simulink model "fdm"  (R2023b)
settings: Solver=VariableStepDiscrete  StartTime=0.0  StopTime=0.02  RelTol=1e-3
libraries: commanapbnd3 x3
settings Model: Creator=RomaW11  LastModifiedBy=RomaW11
settings SolverCC: AlgebraicLoopSolver=TrustRegion
settings DataIOCC: LimitDataPoints=on  SaveOutput=off  SaveTime=off
settings OptimizationCC: BooleanDataType=off  DefaultParameterBehavior=Inlined  LocalBlockOutputs=off  LifeSpan=inf
settings DebuggingCC: AlgebraicLoopMsg=error  SingleTaskRateTransMsg=error  UnconnectedInputMsg=warning  UnconnectedOutputMsg=warning  UnconnectedLineMsg=warning  AllowSymbolicDim=off  SFUnexpectedBacktrackingDiag=warning  SFNoUnconditionalDefaultTransitionDiag=warning  SFExecutionAtInitializationDiag=none  ArithmeticOperatorsInVariantConditions=warning
settings ModelReferenceCC: EnableRefExpFcnMdlSchedulingChecks=on
settings SFSimCC: SimUseLocalCustomCode=off  CustomCodeUndefinedFunction=UseInterfaceOnly
settings RTWCC: RTWUseLocalCustomCode=off
settings CodeAppCC: StateflowObjectComments=on
settings GRTTargetCC: TargetLangStandard=C89/C90 (ANSI)
settings ConfigComp: CovMetricSettings=dw  CovSaveCumulativeToWorkspaceVar=on  CovSaveSingleToWorkspaceVar=on  CovExternalEMLEnable=off  CovSFcnEnable=off

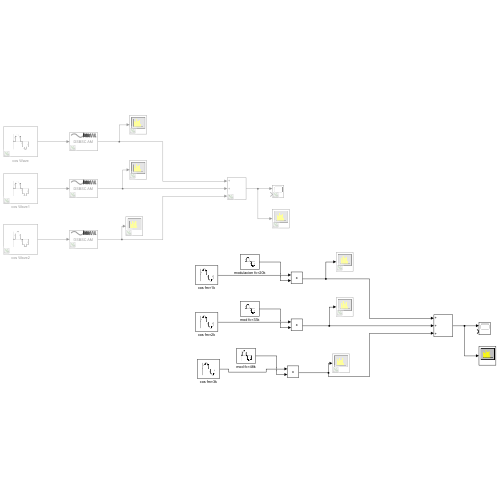
[thumbnail: Simulink's stored preview of the top-level diagram]
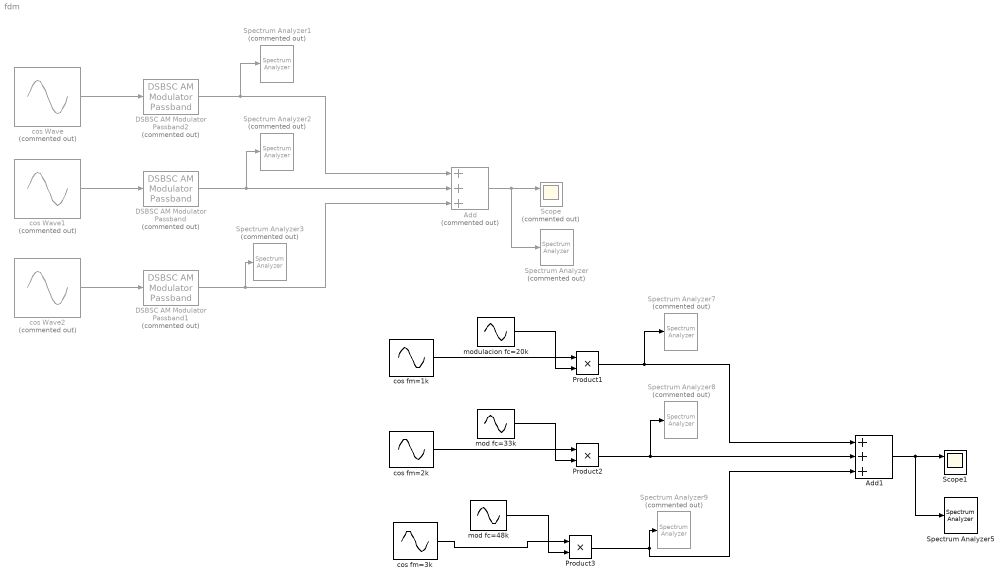
== system fdm ==
  Add : Sum  Commented=on  Inputs=+++
  Add1 : Sum  Inputs=+++
  DSBSC AM Modulator Passband : commanapbnd3/DSBSC AM Modulator Passband  Commented=on  Fc=30000  Ph=0
  DSBSC AM Modulator Passband1 : commanapbnd3/DSBSC AM Modulator Passband  Commented=on  Fc=60000  Ph=0
  DSBSC AM Modulator Passband2 : commanapbnd3/DSBSC AM Modulator Passband  Commented=on  Fc=15000  Ph=0
  Product1 : Product
  Product2 : Product
  Product3 : Product
  Scope : Scope  Commented=on  NumInputPorts=2
  Scope1 : Scope  NumInputPorts=2
  Spectrum Analyzer : SpectrumAnalyzer  Commented=on  WindowPosition=[1.000000,1.000000,1920.000000,1057.000000,]  ScopeFrameLocation=window  SampleRateSource=Property  SampleRate=44.1e3  PlotAsTwoSidedSpectrum=off  FrequencyScale=Log  FrequencySpan=Start and stop frequencies  StartFrequency=20  StopFrequency=20e3  YLimits=[-183.98951359,-66.19382777]
  Spectrum Analyzer1 : SpectrumAnalyzer  Commented=on  WindowPosition=[7.000000,-1079.000000,1920.000000,1057.000000,]  ScopeFrameLocation=window  SampleRateSource=Property  SampleRate=44.1e3  PlotAsTwoSidedSpectrum=off  FrequencyScale=Log  FrequencySpan=Start and stop frequencies  StartFrequency=20  StopFrequency=20e3  YLimits=[-196.41991118,-65.44607318]
  Spectrum Analyzer2 : SpectrumAnalyzer  Commented=on  WindowPosition=[7.000000,-1079.000000,1920.000000,1057.000000,]  ScopeFrameLocation=window  SampleRateSource=Property  SampleRate=44.1e3  PlotAsTwoSidedSpectrum=off  FrequencyScale=Log  FrequencySpan=Start and stop frequencies  StartFrequency=20  StopFrequency=20e3  YLimits=[-195.69141859,-65.14406083]
  Spectrum Analyzer3 : SpectrumAnalyzer  Commented=on  WindowPosition=[7.000000,-1079.000000,1920.000000,1057.000000,]  ScopeFrameLocation=window  SampleRateSource=Property  SampleRate=44.1e3  PlotAsTwoSidedSpectrum=off  FrequencyScale=Log  FrequencySpan=Start and stop frequencies  StartFrequency=20  StopFrequency=20e3  YLimits=[-192.44961022,-65.25345534]
  Spectrum Analyzer5 : SpectrumAnalyzer  WindowPosition=[1.000000,1.000000,1920.000000,1057.000000,]  ScopeFrameLocation=window  SampleRateSource=Property  SampleRate=44.1e3  PlotAsTwoSidedSpectrum=off  FrequencyScale=Log  FrequencySpan=Start and stop frequencies  StartFrequency=20  StopFrequency=20e3  YLimits=[-184.64957668,-66.23917741]  SelectedToolstripTab=spectrumAnalyzerToolstrip.spectralMaskTab
  Spectrum Analyzer7 : SpectrumAnalyzer  Commented=on  WindowPosition=[7.000000,-1079.000000,1920.000000,1057.000000,]  ScopeFrameLocation=window  SampleRateSource=Property  SampleRate=44.1e3  PlotAsTwoSidedSpectrum=off  FrequencyScale=Log  FrequencySpan=Start and stop frequencies  StartFrequency=20  StopFrequency=20e3  YLimits=[-195.69642877,-65.35156214]
  Spectrum Analyzer8 : SpectrumAnalyzer  Commented=on  WindowPosition=[7.000000,-1079.000000,1920.000000,1057.000000,]  ScopeFrameLocation=window  SampleRateSource=Property  SampleRate=44.1e3  PlotAsTwoSidedSpectrum=off  FrequencyScale=Log  FrequencySpan=Start and stop frequencies  StartFrequency=20  StopFrequency=20e3  YLimits=[-193.85684616,-65.21215998]
  Spectrum Analyzer9 : SpectrumAnalyzer  Commented=on  WindowPosition=[7.000000,-1079.000000,1920.000000,1057.000000,]  ScopeFrameLocation=window  SampleRateSource=Property  SampleRate=44.1e3  PlotAsTwoSidedSpectrum=off  FrequencyScale=Log  FrequencySpan=Start and stop frequencies  StartFrequency=20  StopFrequency=20e3  YLimits=[-191.9947139,-65.4940366]
  cos Wave : Sin  Commented=on  Frequency=2*pi*3000  Phase=pi/2  SampleTime=1/300000
  cos Wave1 : Sin  Commented=on  Frequency=2*pi*5000  Phase=pi/2  SampleTime=1/300000
  cos Wave2 : Sin  Commented=on  Frequency=2*pi*7000  Phase=pi/2  SampleTime=1/300000
  cos fm=1k : Sin  Frequency=2*pi*1000  Phase=pi/2  SampleTime=1/300000
  cos fm=2k : Sin  Frequency=2*pi*2000  Phase=pi/2  SampleTime=1/300000
  cos fm=3k : Sin  Frequency=2*pi*3000  Phase=pi/2  SampleTime=1/300000
  mod fc=33k : Sin  Frequency=2*pi*33000  Phase=pi/2  SampleTime=1/300000
  mod fc=48k : Sin  Frequency=2*pi*48000  Phase=pi/2  SampleTime=1/300000
  modulacion fc=20k : Sin  Frequency=2*pi*20000  Phase=pi/2  SampleTime=1/300000
  wires:
  cos Wave/1 -> DSBSC AM Modulator Passband2/1
  cos Wave1/1 -> DSBSC AM Modulator Passband/1
  cos Wave2/1 -> DSBSC AM Modulator Passband1/1
  Add/1 -> Spectrum Analyzer/1, Scope/1
  DSBSC AM Modulator Passband/1 -> Spectrum Analyzer2/1, Add/2
  DSBSC AM Modulator Passband1/1 -> Spectrum Analyzer3/1, Add/3
  DSBSC AM Modulator Passband2/1 -> Spectrum Analyzer1/1, Add/1
  Product1/1 -> Spectrum Analyzer7/1, Add1/1
  Add1/1 -> Spectrum Analyzer5/1, Scope1/1
  Product3/1 -> Add1/3, Spectrum Analyzer9/1
  Product2/1 -> Spectrum Analyzer8/1, Add1/2
  modulacion fc=20k/1 -> Product1/2
  cos fm=1k/1 -> Product1/1
  cos fm=2k/1 -> Product2/1
  mod fc=33k/1 -> Product2/2
  mod fc=48k/1 -> Product3/2
  cos fm=3k/1 -> Product3/1
